simulink model "sustainability_research"  (R2021b)
settings: Solver=VariableStepAuto  StartTime=0.0  StopTime=10.0  RelTol=1e-3
undefined symbols (not defined in the file): K, T_1, T_2
settings Model: Creator=den  LastModifiedBy=den

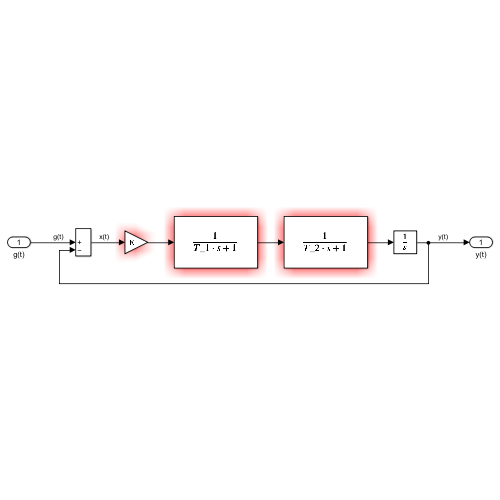
[thumbnail: Simulink's stored preview of the top-level diagram]
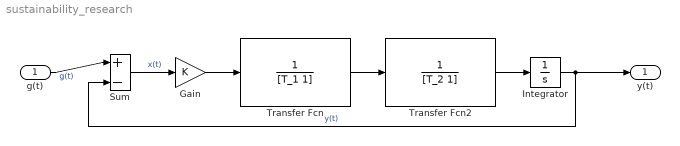
== system sustainability_research ==
  g(t) : Inport
  Gain : Gain  Gain=K
  Integrator : Integrator
  Sum : Sum  Inputs=|+-
  Transfer Fcn : TransferFcn  Denominator=[T_1 1]
  Transfer Fcn2 : TransferFcn  Denominator=[T_2 1]
  y(t) : Outport
  wires:
  Transfer Fcn/1 -> Transfer Fcn2/1
  Gain/1 -> Transfer Fcn/1
  Transfer Fcn2/1 -> Integrator/1
  Integrator/1 -> y(t)/1, Sum/2  "y(t)"
  Sum/1 -> Gain/1  "x(t)"
  g(t)/1 -> Sum/1  "g(t)"
